simulink model "explicit_cruise_planner"  (R2022b)
settings: Solver=FixedStepAuto  StartTime=0.0  StopTime=inf  FixedStep=2.0  RelTol=1e-3
libraries: robotlib x12
settings Model: Creator=ivory  LastModifiedBy=hayat
settings SolverCC: AlgebraicLoopSolver=TrustRegion
settings OptimizationCC: EnhancedBackFolding=on  PassReuseOutputArgsAs=Individual arguments  ZeroExternalMemoryAtStartup=off  ZeroInternalMemoryAtStartup=off  MaxStackSize=64  OptimizeBlockOrder=speed  DifferentSizesBufferReuse=on  OptimizationCustomize=off  EfficientTunableParamExpr=on
settings DebuggingCC: ParameterTunabilityLossMsg=error  UnconnectedInputMsg=warning  UnconnectedOutputMsg=warning  UnconnectedLineMsg=warning  SFMachineParentedDataDiag=warning
settings HardwareCC: ProdBitPerPointer=32  ProdBitPerSizeT=32  ProdBitPerPtrDiffT=32  ProdLargestAtomicFloat=None  ProdIntDivRoundTo=Undefined  ProdEndianess=Unspecified  ProdWordSize=32  ProdHWDeviceType=Generic->Unspecified (assume 32-bit Generic)
settings ModelReferenceCC: EnableRefExpFcnMdlSchedulingChecks=on
settings SFSimCC: MATLABDynamicMemAlloc=off  SimTargetLang=C++
settings RTWCC: Description=Embedded Coder  SystemTargetFile=ert.tlc  HardwareBoard=Robot Operating System (ROS)  TLCOptions="-aInlineSetEventsForThisBaseRateFcn=TLC_FALSE -aSuppressMultiTaskScheduler=TLC_FALSE  -aRateBasedStepFcn=0"  TemplateMakefile=ert_default_tmf  GenerateReport=on  Toolchain=Catkin  IncludeHyperlinkInReport=on  LaunchReport=on  TargetLang=C++  GenerateTraceInfo=on  GenerateTraceReport=on  GenerateTraceReportSl=on  GenerateTraceReportSf=on  GenerateTraceReportEml=on  DLArmComputeVersion=19.05
settings CodeAppCC: ForceParamTrailComments=on  IgnoreCustomStorageClasses=off  OperatorAnnotations=on  SimulinkDataObjDesc=on  SFDataObjDesc=on  InsertBlockDesc=on
settings ERTTargetCC: SupportContinuousTime=on  SupportVariableSizeSignals=on

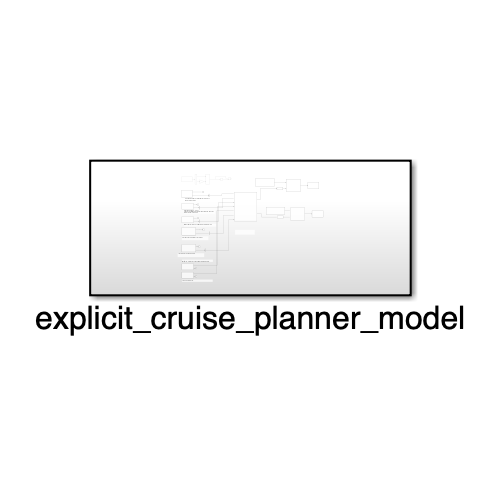
[thumbnail: Simulink's stored preview of the top-level diagram]
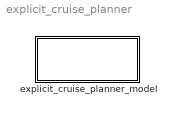
== system explicit_cruise_planner ==
  explicit_cruise_planner_model : Subsystem

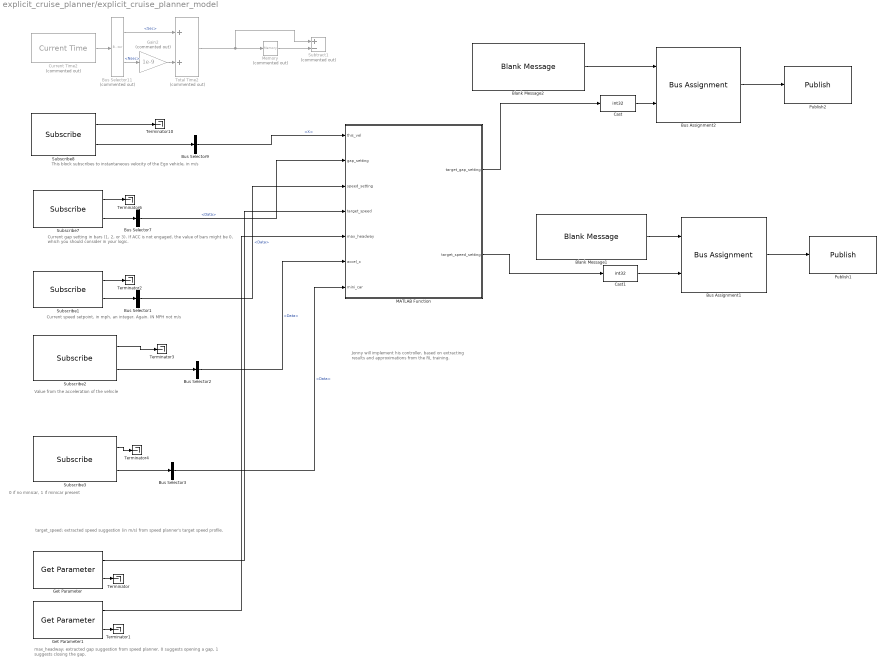
== system explicit_cruise_planner/explicit_cruise_planner_model ==
  note: Jonny will implement his controller, based on extracting results and approximations from the RL training.
  note: Current gap setting in bars (1, 2, or 3).
      | If ACC is not engaged, the value of bars might be 0, which you should consider in your logic.
  note: This block subscribes to instantaneous velocity of the Ego vehicle, in m/s
  note: Current speed setpoint, in mph, an integer. Again. IN MPH not m/s
  note: target_speed: extracted speed suggestion (in m/s) from speed planner's target speed profile.
  note: max_headway: extracted gap suggestion from speed planner.
      | 0 suggests opening a gap, 1 suggests closing the gap.
  note: Value from the acceleration of the vehicle
  note: 0 if no minicar, 1 if minicar present
  Blank Message1 : robotlib/Blank Message  messageClass=Message  entityType=std_msgs/Int32  messageType=std_msgs/Int32  SampleTime=inf  legacyBusStruct=off
  Blank Message2 : robotlib/Blank Message  messageClass=Message  entityType=std_msgs/Int32  messageType=std_msgs/Int32  SampleTime=inf  legacyBusStruct=off
  Bus Assignment1 : BusAssignment  AssignedSignals=Data
  Bus Assignment2 : BusAssignment  AssignedSignals=Data
  Bus Selector{1..3,7} (4 alike) : BusSelector  OutputSignals=Data
  Bus Selector11 : BusSelector  Commented=on  OutputSignals=Sec,Nsec
  Bus Selector9 : BusSelector  OutputSignals=Linear.X
  Cast : DataTypeConversion  OutDataTypeStr=int32  SaturateOnIntegerOverflow=off  RndMeth=Floor
  Cast1 : DataTypeConversion  OutDataTypeStr=int32  SaturateOnIntegerOverflow=off  RndMeth=Floor
  Current Time2 : robotlib/Current Time  Commented=on  OutputFormat=bus  SampleTime=-1  ModelName=microaccel
  Gain2 : Gain  Commented=on  Gain=1e-9
  Get Parameter : robotlib/Get Parameter  ParameterSource=Specify your own  ParameterName=SP_TARGET_SPEED  ParameterType=int32  ParameterMaxArrayLength=16  ParameterInitialValue=70  SampleTime=-1  ShowErrorCodeOutput=on  ModelName=explicit_cruise_planner  BlockId=ParamGet_explicit_cruise_planner_655
  Get Parameter1 : robotlib/Get Parameter  ParameterSource=Specify your own  ParameterName=SP_MAX_HEADWAY  ParameterType=int32  ParameterMaxArrayLength=16  ParameterInitialValue=1  SampleTime=-1  ShowErrorCodeOutput=on  ModelName=explicit_cruise_planner  BlockId=ParamGet_explicit_cruise_planner_657
  MATLAB Function : MATLAB Function  TreatAsAtomicUnit=on
  Memory : Memory  Commented=on
  Publish1 : robotlib/Publish  topicSource=Specify your own  topic=speed_setting  messageType=std_msgs/Int32  legacyBusStruct=off  messageQueueLength=1
  Publish2 : robotlib/Publish  topicSource=Specify your own  topic=gap_setting  messageType=std_msgs/Int32  legacyBusStruct=off  messageQueueLength=1
  Subscribe1 : robotlib/Subscribe  topicSource=Specify your own  topic=speed_setting  messageType=std_msgs/Int32  SampleTime=-1  legacyBusStruct=off  messageQueueLength=1
  Subscribe2 : robotlib/Subscribe  topicSource=Specify your own  topic=accel_x  messageType=std_msgs/Float64  SampleTime=-1  legacyBusStruct=off  messageQueueLength=1
  Subscribe3 : robotlib/Subscribe  topicSource=Specify your own  topic=mini_car  messageType=std_msgs/Int32  SampleTime=-1  legacyBusStruct=off  messageQueueLength=1
  Subscribe7 : robotlib/Subscribe  topicSource=Specify your own  topic=gap_setting  messageType=std_msgs/Int32  SampleTime=-1  legacyBusStruct=off  messageQueueLength=1
  Subscribe8 : robotlib/Subscribe  topicSource=Specify your own  topic=vel  messageType=geometry_msgs/Twist  SampleTime=-1  legacyBusStruct=off  messageQueueLength=1
  Subtract1 : Sum  Commented=on  Inputs=+-
  Terminator{,1..4,6,10} (7 alike) : Terminator
  Total Time2 : Sum  Commented=on
  wires:
  Bus Selector11/1 -> Total Time2/1  "<Sec>"
  Gain2/1 -> Total Time2/2
  Bus Selector11/2 -> Gain2/1  "<Nsec>"
  Total Time2/1 -> Subtract1/1, Memory/1
  Current Time2/1 -> Bus Selector11/1
  Memory/1 -> Subtract1/2
  Subscribe8/2 -> Bus Selector9/1
  Subscribe8/1 -> Terminator10/1
  Bus Selector9/1 -> MATLAB Function/1(this_vel)  "<X>"
  Subscribe7/1 -> Terminator6/1
  Subscribe7/2 -> Bus Selector7/1
  Get Parameter/1 -> MATLAB Function/4(target_speed)
  Get Parameter/2 -> Terminator/1
  Get Parameter1/2 -> Terminator1/1
  Get Parameter1/1 -> MATLAB Function/5(max_headway)
  Bus Assignment2/1 -> Publish2/1
  Blank Message2/1 -> Bus Assignment2/1
  MATLAB Function/1(target_gap_setting) -> Cast/1
  Blank Message1/1 -> Bus Assignment1/1
  Bus Assignment1/1 -> Publish1/1
  Cast/1 -> Bus Assignment2/2
  Cast1/1 -> Bus Assignment1/2
  Subscribe1/1 -> Terminator2/1
  Subscribe1/2 -> Bus Selector1/1
  Bus Selector1/1 -> MATLAB Function/3(speed_setting)  "<Data>"
  MATLAB Function/2(target_speed_setting) -> Cast1/1
  Bus Selector7/1 -> MATLAB Function/2(gap_setting)  "<Data>"
  Bus Selector2/1 -> MATLAB Function/6(accel_x)  "<Data>"
  Subscribe2/2 -> Bus Selector2/1
  Subscribe2/1 -> Terminator3/1
  Bus Selector3/1 -> MATLAB Function/7(mini_car)  "<Data>"
  Subscribe3/1 -> Terminator4/1
  Subscribe3/2 -> Bus Selector3/1

== matlab function explicit_cruise_planner/explicit_cruise_planner_model/MATLAB Function ==
  settings: updateMethod=DISCRETE
  data: this_vel input; gap_setting input; speed_setting input; target_gap_setting output; target_speed input; max_headway input; target_speed_setting output; accel_x input; mini_car input
function [target_gap_setting, target_speed_setting] =  get_acc_values(this_vel, gap_setting, speed_setting, ...
            target_speed, max_headway, accel_x, mini_car)
        %%"""See parent class."""
        % TODO (Amaury): replace with your controller's logic
        MPH_TO_MS = 0.44704;
        history_speed = NaN;
        with_inrix = true;
        vdes_n_avg = 640;
        vdes_scaling = 1.2;
        catch_up_intensity = 1.1;
        weight = 0.8;
        inrix_scaling = 1.1;
        vmax = 30;
        strong_guide = false;

        persistent prev_ego_vels

        %Store previous ego vel
        if isempty(prev_ego_vels)
            prev_ego_vels = zeros(1,vdes_n_avg);
            prev_ego_vels(end) = this_vel;
        else
            prev_ego_vels = [prev_ego_vels(2:end),this_vel];
        end

        
        spd_err = (speed_setting * MPH_TO_MS) - this_vel;
        if spd_err > 0.6
            k = 0.5; % TODO: change to params['p20']
            c = 0; % TODO: change to params['p21']
            max_accel = 1.0; % TODO: change to params['p3']
            spd_control_accel = min([max_accel, k * spd_err + c]);
        else
            k = 0.4; % TODO: change to params['p22']
            c = 0; % TODO: change to params['p23']
            min_accel = -1.0; % TODO: change to params['p3']
            spd_control_accel = max([min_accel, k * spd_err + c]);
        end

        if accel_x == None
            accel_delta = 0;
            accel_x = 0;
        else
            accel_delta = spd_control_accel - accel_x;
        end

        if target_speed == -1 | ~with_inrix % no speed planner
           v_des_no_data = vdes_scaling * mean(prev_ego_vels(end-vdes_n_avg : end));
            if ~isnan(history_speed) % historic guide available
                v_des_no_data = max(min(v_des_no_data, 1.2 * history_speed), 0.8 * history_speed);
            end
           target_speed_setting = v_des_no_data;

           if strong_guide && ~isnan(history_speed)
               target_speed_setting = min(1.2 * history_speed, target_speed_setting);
           end
        else % with speed planner
            if accel_delta <= 0.1  % leader barely influencing our speed
                target_speed_setting = min([speed_setting * MPH_TO_MS, target_speed * inrix_scaling]);
            else  % leader strongly influencing our speed
                target_speed_setting = target_speed;
            end
        end

        if mini_car == 0% no car in sight, go faster
            target_speed_setting = min([(speed_setting + 1) * MPH_TO_MS, target_speed_setting * catch_up_intensity]);
        end

%         if mini_car == 0  % no car in sight, go faster
%             target_speed_setting = min([(speed_setting + 1) * MPH_TO_MS, target_speed * 1.2]);
%         else
%             if accel_delta <= 0.1  % leader barely influencing our speed
%                 target_speed_setting = min([speed_setting * MPH_TO_MS, target_speed * 1.1]);
%             else  % leader strongly influencing our speed
%                 target_speed_setting = target_speed;
%             end
%         end

        if max_headway == 1
            if this_accel < -1
                target_gap_setting = max([gap_setting - 1, 1]);
            elseif accel_x > 0.5
                target_gap_setting = 3;
            else
                target_gap_setting = max([gap_setting, 1]);
            end
        else
            target_gap_setting = 3;
        end

        % convert to int MPH in [20, 80]
        target_speed_setting = int32(round(target_speed_setting / MPH_TO_MS));
        target_speed_setting = min([max([target_speed_setting, 20]), 80]);

end
